simulink model "IncreaseButtonHarness"  (R2022b)
settings: Solver=FixedStepDiscrete  StartTime=0.0  StopTime=10  FixedStep=0.1  RelTol=1e-3  EnableMultiTasking=on
settings Model: Creator=graziaferrara  LastModifiedBy=graziaferrara
settings SolverCC: AlgebraicLoopSolver=TrustRegion  AutoInsertRateTranBlk=on
settings DataIOCC: LimitDataPoints=on
settings OptimizationCC: LifeSpan=inf
settings DebuggingCC: UnconnectedInputMsg=warning  UnconnectedOutputMsg=warning  UnconnectedLineMsg=warning  AllowSymbolicDim=off  SFUnexpectedBacktrackingDiag=warning  SFNoUnconditionalDefaultTransitionDiag=warning  SFExecutionAtInitializationDiag=none  ArithmeticOperatorsInVariantConditions=warning
settings ModelReferenceCC: EnableRefExpFcnMdlSchedulingChecks=on
settings SFSimCC: SimUseLocalCustomCode=off  CustomCodeUndefinedFunction=UseInterfaceOnly
settings RTWCC: RTWUseLocalCustomCode=off  DLArmComputeVersion=19.05
settings CodeAppCC: StateflowObjectComments=on
settings GRTTargetCC: TargetLangStandard=C89/C90 (ANSI)
settings ConfigComp: CovEnable=on  RecordCoverage=on  CovMetricSettings=dw  CovEnableCumulative=off  CovSaveCumulativeToWorkspaceVar=on  CovSaveSingleToWorkspaceVar=on  CovModelRefEnable=on  CovExternalEMLEnable=off  CovSFcnEnable=off  DVTestSuiteOptimization=Auto  DVDetectOutOfBounds=on  DVModelReferenceHarness=on  DVHarnessSource=Signal Editor

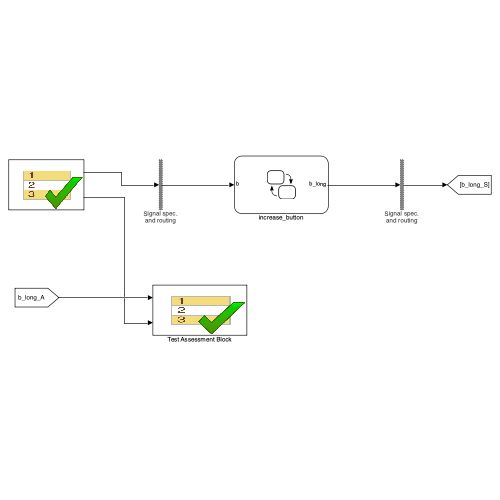
[thumbnail: Simulink's stored preview of the top-level diagram]
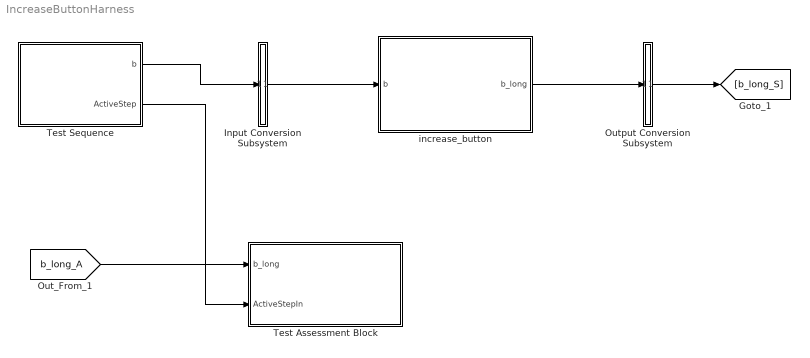
== system IncreaseButtonHarness ==
  Input Conversion Subsystem : Subsystem  Tag=__SLT_ICS__  Description=|
      | Signal spec.
      | and routing
      settings: AttributesFormatString=%<Description>
  Output Conversion Subsystem : Subsystem  Tag=__SLT_OCS__  Description=|
      | Signal spec.
      | and routing
      settings: AttributesFormatString=%<Description>
  Test Assessment Block : Test Sequence  Tag=__SLT_ASMT__  TreatAsAtomicUnit=on
  Test Sequence : Test Sequence  TreatAsAtomicUnit=on
  increase_button : Stateflow chart  TreatAsAtomicUnit=on
  wires:
  Test Sequence/1(b) -> Input Conversion Subsystem/1(Inport_1)
  Output Conversion Subsystem/1(Outport_1) -> [b_long_S]
  Input Conversion Subsystem/1(Outport_1) -> increase_button/1(b)
  increase_button/1(b_long) -> Output Conversion Subsystem/1(Inport_1)
  [b_long_A] -> Test Assessment Block/1(b_long)
  Test Sequence/2(ActiveStep) -> Test Assessment Block/2(ActiveStepIn)

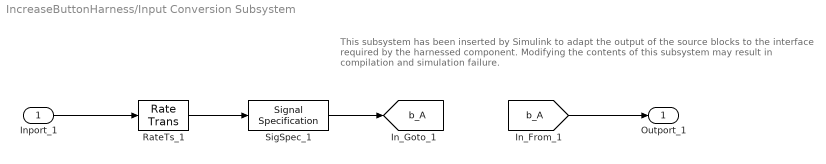
== system IncreaseButtonHarness/Input Conversion Subsystem ==
  note: This subsystem has been inserted by Simulink to adapt the output of the source blocks to the interface required by the harnessed component.
      |  Modifying the contents of this subsystem may result in compilation and simulation failure.
  Inport_1 : Inport
  RateTs_1 : RateTransition  OutPortSampleTime=[-1, 0]
  SigSpec_1 : SignalSpecification  OutDataTypeStr=boolean  Dimensions=[1]  SampleTime=[-1, 0]
  Outport_1 : Outport
  tag scope: b_A=global
  wires:
  [b_A] -> Outport_1/1
  SigSpec_1/1 -> [b_A]
  RateTs_1/1 -> SigSpec_1/1
  Inport_1/1 -> RateTs_1/1

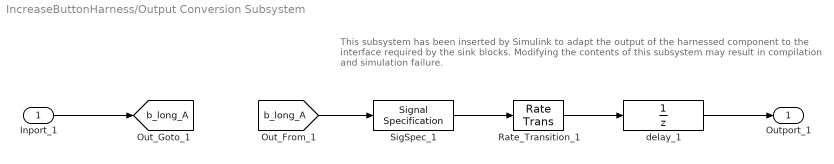
== system IncreaseButtonHarness/Output Conversion Subsystem ==
  note: This subsystem has been inserted by Simulink to adapt the output of the harnessed component to the interface required by the sink blocks.
      |  Modifying the contents of this subsystem may result in compilation and simulation failure.
  Inport_1 : Inport
  Rate_Transition_1 : RateTransition  OutPortSampleTimeOpt=Inherit
  SigSpec_1 : SignalSpecification  OutDataTypeStr=boolean  Dimensions=[1]  SampleTime=0.1
  delay_1 : UnitDelay  SampleTime=-1
  Outport_1 : Outport
  tag scope: b_long_A=global
  wires:
  Inport_1/1 -> [b_long_A]
  [b_long_A] -> SigSpec_1/1
  SigSpec_1/1 -> Rate_Transition_1/1
  Rate_Transition_1/1 -> delay_1/1
  delay_1/1 -> Outport_1/1

== stateflow chart IncreaseButtonHarness/Test Assessment Block ==
  state CorrectBehavior
    state Run
      settings: description=Esecuzione test
      state Verify_CB_Init
        verify(b_long == 1);
        settings: description=Bottone inizialmente non premuto.
      state Verify_CB_ButtonPressed
        settings: description=Bottone premuto
        state Verify_CB_ButtonPressed_1
          verify(b_long == 1);
          settings: description=Fino a che non passa 1 secondo, non viene rilevato alcun cambiamento nella potenza.
        state Verify_CB_ButtonPressed_2
          verify(b_long == 0);
          settings: description=Viene rilevata la pressione lunga.
        (default) -> Verify_CB_ButtonPressed_1
        Verify_CB_ButtonPressed_1 -> Verify_CB_ButtonPressed_2 : [
            | after(1,sec)
            | ]
      state step_1_2
      (default) -> (junction 105)
      CorrectBehavior.Run -> (junction 105)
      (junction 105) -> (junction 106) [order 1] : [ActiveStepIn == ActiveStepEnumH1.CB_Init
          | ]
      (junction 106) -> Verify_CB_Init [order 1] : [~in(CorrectBehavior.Run.Verify_CB_Init)]
      (junction 105) -> (junction 114) [order 2]
      (junction 106) -> (junction 109) [order 2]
      (junction 114) -> (junction 115) [order 1] : [ActiveStepIn == ActiveStepEnumH1.CB_ButtonPressed
          | ]
      (junction 115) -> Verify_CB_ButtonPressed [order 1] : [~in(CorrectBehavior.Run.Verify_CB_ButtonPressed)]
      (junction 114) -> (junction 136) [order 2]
      (junction 115) -> (junction 118) [order 2]
      (junction 136) -> (junction 137)
      (junction 137) -> CorrectBehavior.Run.step_1_2 [order 1] : [~in(CorrectBehavior.Run.step_1_2)]
      (junction 137) -> (junction 140) [order 2]
    (default) -> CorrectBehavior.Run
  state EarlyRelease
    state Run
      settings: description=Esecuzione test
      state Verify_ER_Init
        verify(b_long == 1);
        settings: description=Inizialmente il pulsante non è premuto.
      state Verify_ER_ButtonPressed
        verify(b_long == 1);
        settings: description=Viene premuto il pulsante, ma non per un tempo sufficientemente lungo da richiedere un cambio potenza.
      state Verify_ER_ButtonReleased
        verify(b_long == 1);
        settings: description=Quando il pulsante viene rilasciato (prima di un secondo, perché abbiamo scelto 0.5), la pressione lunga non viene rilevata.
      state step_1_2
      EarlyRelease.Run -> (junction 234)
      (default) -> (junction 234)
      (junction 234) -> (junction 235) [order 1] : [ActiveStepIn == ActiveStepEnumH1.ER_Init
          | ]
      (junction 235) -> Verify_ER_Init [order 1] : [~in(EarlyRelease.Run.Verify_ER_Init)]
      (junction 234) -> (junction 243) [order 2]
      (junction 235) -> (junction 238) [order 2]
      (junction 243) -> (junction 244) [order 1] : [ActiveStepIn == ActiveStepEnumH1.ER_ButtonPressed
          | ]
      (junction 244) -> Verify_ER_ButtonPressed [order 1] : [~in(EarlyRelease.Run.Verify_ER_ButtonPressed)]
      (junction 243) -> (junction 258) [order 2]
      (junction 244) -> (junction 247) [order 2]
      (junction 258) -> (junction 259) [order 1] : [ActiveStepIn == ActiveStepEnumH1.ER_ButtonReleased
          | ]
      (junction 259) -> Verify_ER_ButtonReleased [order 1] : [~in(EarlyRelease.Run.Verify_ER_ButtonReleased)]
      (junction 258) -> (junction 266) [order 2]
      (junction 259) -> (junction 262) [order 2]
      (junction 266) -> (junction 267)
      (junction 267) -> EarlyRelease.Run.step_1_2 [order 1] : [~in(EarlyRelease.Run.step_1_2)]
      (junction 267) -> (junction 270) [order 2]
    (default) -> EarlyRelease.Run
  state General
    state Run
      settings: description=Esecuzione test
      state Verify_G_Init
        verify(b_long == 1);
        settings: description=Inizialmente il bottone è rilasciato, per cui non è stato rilevato alcun long press.
      state Verify_G_ButtonPressed1
        settings: description=Bottone premuto
        state Verify_G_ButtonPressed1_1
          verify(b_long == 1);
          settings: description=Fino a che non passa 1 secondo, non viene rilevato alcun cambiamento nella potenza.
        state Verify_G_ButtonPressed1_2
          verify(b_long == 0);
          settings: description=Viene rilevata la pressione lunga.
        (default) -> Verify_G_ButtonPressed1_1
        Verify_G_ButtonPressed1_1 -> Verify_G_ButtonPressed1_2 : [
            | after(1,sec)
            | ]
      state Verify_G_ButtonReleased
        verify(b_long == 1);
        settings: description=La pressione lunga viene resettata.
      state Verify_G_ButtonPressed2
        settings: description=Bottone premuto
        state Verify_G_ButtonPressed2_1
          verify(b_long == 1)
          settings: description=Fino a che non passa 1 secondo, non viene rilevato alcun cambiamento nella potenza.
        state Verify_G_ButtonPressed2_2
          verify(b_long == 0);
          settings: description=Viene rilevata la pressione lunga.
        state Verify_G_ButtonPressed2_3
          verify(b_long == 1)
          settings: description=La pressione lunga viene resettata.
        (default) -> Verify_G_ButtonPressed2_1
        Verify_G_ButtonPressed2_1 -> Verify_G_ButtonPressed2_2 : [
            | after(1,sec)
            | ]
        Verify_G_ButtonPressed2_2 -> Verify_G_ButtonPressed2_3 : [
            | after(sampleTime,sec)
            | ]
      state Verify_G_ButtonReleased2
        verify(b_long == 1)
        settings: description=Il bottone è rilasciato, per cui non viene rilevato alcun long press
      state step_1_2
      (default) -> (junction 311)
      General.Run -> (junction 311)
      (junction 311) -> (junction 312) [order 1] : [ActiveStepIn == ActiveStepEnumH1.G_Init
          | ]
      (junction 312) -> Verify_G_Init [order 1] : [~in(General.Run.Verify_G_Init)]
      (junction 311) -> (junction 320) [order 2]
      (junction 312) -> (junction 315) [order 2]
      (junction 320) -> (junction 321) [order 1] : [ActiveStepIn == ActiveStepEnumH1.G_ButtonPressed
          | ]
      (junction 321) -> Verify_G_ButtonPressed1 [order 1] : [~in(General.Run.Verify_G_ButtonPressed1)]
      (junction 320) -> (junction 335) [order 2]
      (junction 321) -> (junction 324) [order 2]
      (junction 335) -> (junction 336) [order 1] : [ActiveStepIn == ActiveStepEnumH1.G_ButtonReleased
          | ]
      (junction 336) -> Verify_G_ButtonReleased [order 1] : [~in(General.Run.Verify_G_ButtonReleased)]
      (junction 335) -> (junction 343) [order 2]
      (junction 336) -> (junction 339) [order 2]
      (junction 343) -> (junction 344) [order 1] : [ActiveStepIn == ActiveStepEnumH1.G_ButtonPressed2
          | ]
      (junction 344) -> Verify_G_ButtonPressed2 [order 1] : [~in(General.Run.Verify_G_ButtonPressed2)]
      (junction 343) -> (junction 384) [order 2]
      (junction 344) -> (junction 347) [order 2]
      (junction 384) -> (junction 385) [order 1] : [ActiveStepIn == ActiveStepEnumH1.G_ButtonReleased2
          | ]
      (junction 385) -> Verify_G_ButtonReleased2 [order 1] : [~in(General.Run.Verify_G_ButtonReleased2)]
      (junction 384) -> (junction 351) [order 2]
      (junction 385) -> (junction 388) [order 2]
      (junction 351) -> (junction 352)
      (junction 352) -> General.Run.step_1_2 [order 1] : [~in(General.Run.step_1_2)]
      (junction 352) -> (junction 355) [order 2]
    (default) -> General.Run
  state LateRelease
    state Run
      settings: description=Esecuzione test
      state Verify_LR_Init
        verify(b_long == 1);
        settings: description=Inizialmente il pulsante non è premuto.
      state Verify_LR_ButtonPressed
        settings: description=Viene premuto il pulsante.
        state Verify_LR_ButtonPressed_1
          verify(b_long == 1);
          settings: description=Fino a che non passa 1 secondo, non viene rilevato alcun cambiamento nella potenza.
        state Verify_LR_ButtonPressed_2
          verify(b_long == 0);
          settings: description=Viene rilevata la pressione lunga.
        state Verify_LR_ButtonPressed_3
          verify(b_long == 1);
          settings: description=La pressione lunga viene resettata.
        (default) -> Verify_LR_ButtonPressed_1
        Verify_LR_ButtonPressed_1 -> Verify_LR_ButtonPressed_2 : [
            | after(1,sec)
            | ]
        Verify_LR_ButtonPressed_2 -> Verify_LR_ButtonPressed_3 : [
            | after(sampleTime,sec)
            | ]
      state Verify_LR_ButtonReleased
        verify(b_long == 1);
        settings: description=Quando il pulsante viene rilasciato la pressione lunga non è verificata.
      state step_1_2
      (junction 471) -> (junction 474) [order 2]
      (junction 462) -> (junction 470) [order 2]
      LateRelease.Run -> (junction 445)
      (default) -> (junction 445)
      (junction 445) -> (junction 446) [order 1] : [ActiveStepIn == ActiveStepEnumH1.LR_Init
          | ]
      (junction 446) -> Verify_LR_Init [order 1] : [~in(LateRelease.Run.Verify_LR_Init)]
      (junction 445) -> (junction 454) [order 2]
      (junction 446) -> (junction 449) [order 2]
      (junction 454) -> (junction 455) [order 1] : [ActiveStepIn == ActiveStepEnumH1.LR_ButtonPressed
          | ]
      (junction 455) -> Verify_LR_ButtonPressed [order 1] : [~in(LateRelease.Run.Verify_LR_ButtonPressed)]
      (junction 454) -> (junction 462) [order 2]
      (junction 455) -> (junction 458) [order 2]
      (junction 462) -> (junction 463) [order 1] : [ActiveStepIn == ActiveStepEnumH1.LR_ButtonReleased
          | ]
      (junction 463) -> Verify_LR_ButtonReleased [order 1] : [~in(LateRelease.Run.Verify_LR_ButtonReleased)]
      (junction 463) -> (junction 466) [order 2]
      (junction 470) -> (junction 471)
      (junction 471) -> LateRelease.Run.step_1_2 [order 1] : [~in(LateRelease.Run.step_1_2)]
    (default) -> LateRelease.Run
  (default) -> CorrectBehavior [order 1] : [Active_Scenario_Index == 1]
  (default) -> EarlyRelease [order 2] : [Active_Scenario_Index == 2]
  (default) -> General [order 3] : [Active_Scenario_Index == 3]
  (default) -> LateRelease [order 4] : {assert(Active_Scenario_Index == 4,'The value of Scenario Parameter ''Active_Scenario_Index'' is not valid. Use the index of the scenario to specify it.')}
  data: b_long input boolean size=[1]; ActiveStepIn input; Active_Scenario_Index parameter =3; sampleTime constant double =str2num(get_param('Team3_InductionCooker','FixedStep'))

== stateflow chart IncreaseButtonHarness/increase_button ==
  note: Bottone a livelli, la pressione per un numero di secondi pari a DURATION permette di avere un uscita alta in maniera istantanea.
      | Per avere in output un valore PRESSED, è necessare lasciare il bottone e premere tra un output e l'altro.
  state Wait
    en: b_long = RELEASED
  state Pressed
    en: b_long = RELEASED;
    on after(DURATION,sec): b_long = PRESSED
  state LongPressed
    en: b_long = RELEASED
  (default) -> Wait
  Wait -> Pressed : [b == PRESSED]
  Pressed -> Wait [order 1] : [b == RELEASED]
  LongPressed -> Wait : [b == RELEASED]
  Pressed -> LongPressed [order 2] : [b_long == PRESSED && b == PRESSED]
  data: b_long output boolean size=1; PRESSED constant boolean size=1 =0; RELEASED constant boolean size=1 =1; b input boolean size=1; DURATION constant double size=1 =1

== stateflow chart IncreaseButtonHarness/Test Sequence ==
  settings: updateMethod=DISCRETE  sampleTime=0.1
  state CorrectBehavior
    state CB_Init
      %% Initialize data outputs.
      b = true;
      settings: description=|
          | Pulsante non premuto.
          | Il pulsante lavora in logica negata come avviene per il bottone presente sulla scheda.
    state CB_ButtonPressed
      b = false
      settings: description=|
          | Pulsante premuto.
          | Consideriamo questo step attivo per 1 secondo.
          | Attiva la transizione da Wait a Pressed.
    state CB_ButtonReleased
      b = true
      settings: description=|
          | Pulsante rilasciato.
          | Ci aspettiamo che sia stata rilevata la richiesta di aumento della potenza.
          | Il pulsante torna nello stato di Wait, attivando la transizione da Pressed a Wait.
    (default) -> CB_Init
    CB_Init -> CB_ButtonPressed : [
        | true
        | ]
    CB_ButtonPressed -> CB_ButtonReleased : [
        | after(1+ sampleTime,sec)
        | ]
  state EarlyRelease
    state ER_Init
      %% Initialize data outputs.
      b = true;
      settings: description=|
          | Pulsante non premuto.
          | Il pulsante lavora in logica negata come avviene per il bottone presente sulla scheda.
    state ER_ButtonPressed
      b = false
      settings: description=|
          | Pulsante premuto.
          | Lo stato passa da Wait a Pressed.
          | Consideriamo questo step attivo per meno di 1 secondo (ad esempio mezzo secondo).
    state ER_ButtonReleased
      b = true
      settings: description=|
          | Pulsante rilasciato dopo mezzo secondo.
          | Lo stato passa da Pressed a Wait.
          | Ci aspettiamo che non sia stata rilevata la richiesta di aumento della potenza.
    (default) -> ER_Init
    ER_Init -> ER_ButtonPressed : [
        | true
        | ]
    ER_ButtonPressed -> ER_ButtonReleased : [
        | after(0.5,sec)
        | ]
  state General
    state G_Init
      %% Initialize data outputs.
      b = true;
      settings: description=|
          | Pulsante non premuto.
          | Il pulsante lavora in logica negata come avviene per il bottone presente sulla scheda.
    state G_ButtonPressed
      b = false
      settings: description=|
          | Pulsante premuto.
          | Consideriamo questo step attivo per 1 secondo.
          | Attiva la transizione da Wait a Pressed.
    state G_ButtonReleased
      b = true
      settings: description=|
          | Pulsante rilasciato.
          | Ci aspettiamo che sia stata rilevata la richiesta di aumento della potenza.
          | Il pulsante torna nello stato di Wait, attivando la transizione da Pressed a Wait.
    state G_ButtonPressed2
      b = false
      settings: description=|
          | Pulsante premuto a lungo.
          | Prima passa da Wait a Pressed e poi da Pressed a LongPressed.
    state G_ButtonReleased2
      b = true
      settings: description=|
          | Pulsante rilasciato.
          | Passa da LongPressed a Wait.
    (default) -> G_Init
    G_Init -> G_ButtonPressed : [
        | true
        | ]
    G_ButtonPressed -> G_ButtonReleased : [
        | after(1+ sampleTime,sec)
        | ]
    G_ButtonReleased -> G_ButtonPressed2 : [
        | after(0.1,sec)
        | ]
    G_ButtonPressed2 -> G_ButtonReleased2 : [
        | after(2+ sampleTime,sec)
        | ]
  state LateRelease
    state LR_Init
      %% Initialize data outputs.
      b = true;
      settings: description=|
          | Pulsante non premuto.
          | Il pulsante lavora in logica negata come avviene per il bottone presente sulla scheda.
    state LR_ButtonPressed
      b = false
      settings: description=|
          | Pulsante premuto.
          | Lo stato passa da Wait a Pressed e da Pressed a LongPressed.
          | Consideriamo questo step attivo per più di 1 secondo (ad esempio un secondo e mezzo).
    state LR_ButtonReleased
      b = true
      settings: description=|
          | Pulsante rilasciato dopo un secondo e mezzo.
          | Lo stato passa da LongPressed a Wait.
    (default) -> LR_Init
    LR_Init -> LR_ButtonPressed : [
        | true
        | ]
    LR_ButtonPressed -> LR_ButtonReleased : [
        | after(1.5,sec)
        | ]
  (default) -> CorrectBehavior [order 1] : [Active_Scenario_Index == 1]
  (default) -> EarlyRelease [order 2] : [Active_Scenario_Index == 2]
  (default) -> General [order 3] : [Active_Scenario_Index == 3]
  (default) -> LateRelease [order 4] : {assert(Active_Scenario_Index == 4,'The value of Scenario Parameter ''Active_Scenario_Index'' is not valid. Use the index of the scenario to specify it.')}
  data: b output boolean size=[1]; ActiveStep output Enum: ActiveStepEnumH1; sampleTime constant double =str2num(get_param('Team3_InductionCooker','FixedStep')); Active_Scenario_Index parameter =3
